simulink model "dynamic_simulation_control"  (R2020b)
settings: Solver=FixedStepAuto  StartTime=time_start  StopTime=time_end  FixedStep=dt  RelTol=1e-3
values from neighbouring files (symbols this model uses):
  B_env = [0;10;0]    [init_dynamic_sim.m]
  dth0 = [0; 0; 0]    [dynamic_simulation.m]    (also in init_dynamic_sim.m = dq0)
  dv = 1e-2    (= 0.01)    [Fs_3DOF.m]    (also in init_dynamic_sim.m)
  Fc = Fs    [Fs_3DOF.m]    (also in init_dynamic_sim.m)
  filt_den = [1/w0^2 2*xi/w0 1]    [init_dynamic_sim.m]
  filt_num = 1    [init_dynamic_sim.m]
  Fs = zeros(3,1)    [DynModel_3DOF.m]    (also in Fs_3DOF.m = [0.97571; 0.65131; 0.25819]; InvDynModel_3DOF.m; init_dynamic_sim.m = [0.97571; 0.65131; 0.25819])
  Fv = zeros(3,3)    [DynModel_3DOF.m]    (also in InvDynModel_3DOF.m; init_dynamic_sim.m = diag([0.5,0.37,0.7]))
  fz0 = 0    [init_dynamic_sim.m]
  K = 0.015    [init_dynamic_sim.m]
  K_env = [0;100;0]    [init_dynamic_sim.m]
  Ki = 0.08    [init_dynamic_sim.m]
  Kj = [1;1;1]*5    [init_dynamic_sim.m]
  Kjd = [1;1;1]*0.1    [init_dynamic_sim.m]
  Kv = [2500;1500;2000]/256    [init_dynamic_sim.m]
  Kvi = [3000;900;1000]/65536    [init_dynamic_sim.m]
  Kx = [20;0;0]    [init_dynamic_sim.m]
  Kxi = [0;0;0]    [init_dynamic_sim.m]
  M_env = [0;1;0]    [init_dynamic_sim.m]
  nu = nu.*eye(3)    [DynModel_3DOF.m]    (also in InvDynModel_3DOF.m; init_dynamic_sim.m = [0.65;0.65;0.65])
  R = [156;100;71]    [init_dynamic_sim.m]
  ry0 = acos(r(1,1))    [init_dynamic_sim.m]
  Tc = [0.0335;0.0335;0.051]    [init_dynamic_sim.m]
  th0 = 0    [DGM_youBot.m]    (also in DGM_youBot_sym.m; dynamic_simulation.m = q_dh - (q0_kuka - q_rob); init_dynamic_sim.m = theta_DH(2:4) - (q0 - KUKA_offset(2:4)))
  thmax = theta_DH - (qmin - KUKA_offset)    [init_dynamic_sim.m]
  thmin = theta_DH - (qmax - KUKA_offset)    [init_dynamic_sim.m]
  x0 = p0(1)    [init_dynamic_sim.m]    (also in jacobian_computation.m = 0.033)
  z0 = 0.3    [dynamic_simulation.m]    (also in init_dynamic_sim.m = p0(3); jacobian_computation.m = 0.147)
undefined symbols (not defined in the file or in its folder): p0
libraries: aerolibutil x1, simulink x1
settings Model: Creator=fortineau_vin  LastModifiedBy=fortineau_vin
settings DataIOCC: ReturnWorkspaceOutputs=off
settings DebuggingCC: ArithmeticOperatorsInVariantConditions=warning
settings SFSimCC: SimUseLocalCustomCode=off  CustomCodeUndefinedFunction=UseInterfaceOnly
settings RTWCC: RTWUseLocalCustomCode=off

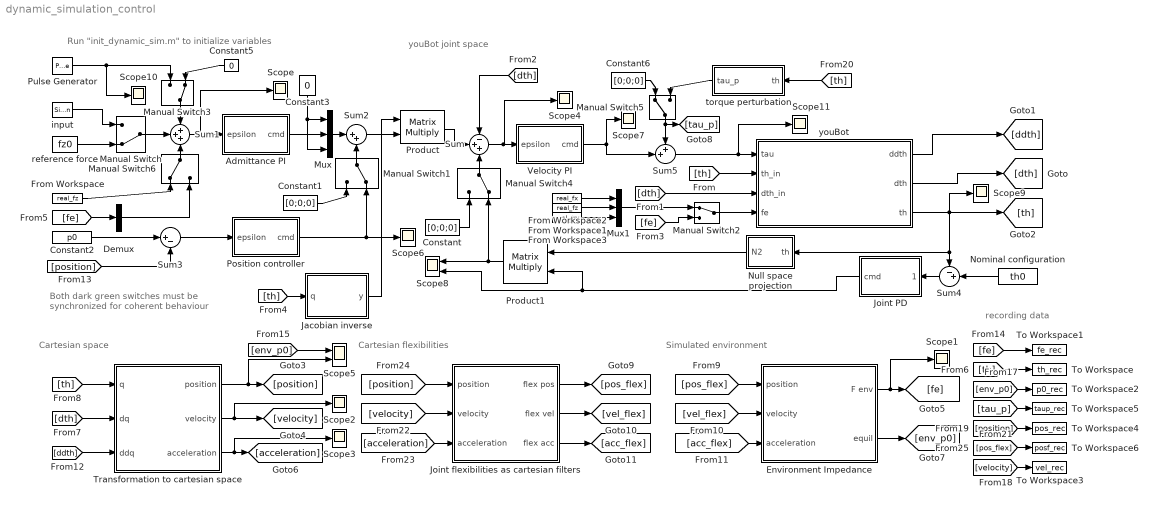
== system dynamic_simulation_control ==
  note: Both dark green switches must
      | be synchronized for coherent behaviour
  note: recording data
  note: Run "init_dynamic_sim.m" to initialize variables
  note: youBot joint space
  note: Simulated environment
  note: Cartesian flexibilities
  note: Cartesian space
  Admittance PI : Subsystem
  Constant : Constant  Value=[0;0;0]
  Constant1 : Constant  Value=[0;0;0]
  Constant2 : Constant  Value=p0
  Constant3 : Constant  Value=0
  Constant5 : Constant  Value=0
  Constant6 : Constant  Value=[0;0;0]
  Demux : Demux  Outputs=3
  "Environment Impedance " : Subsystem
  From Workspace : FromWorkspace  VariableName=real_fz
  From Workspace1 : FromWorkspace  VariableName=real_fz
  From Workspace2 : FromWorkspace  VariableName=real_fx
  From Workspace3 : FromWorkspace  VariableName=real_fry
  Jacobian inverse : MATLAB Function  TreatAsAtomicUnit=on
  Joint PD : Subsystem
  Joint flexibilities as cartesian filters : Subsystem
  Manual Switch{,1,3..4} (4 alike) : ManualSwitch  CurrentSetting=0
  Manual Switch2 : ManualSwitch
  Manual Switch5 : ManualSwitch
  Manual Switch6 : ManualSwitch
  Mux : Mux  Inputs=3
  Mux1 : Mux  Inputs=3
  Nominal configuration : Constant  Value=th0
  Null space projection : Subsystem
  Position controller : Subsystem
  Product : Product  Multiplication=Matrix(*)
  Product1 : Product  Multiplication=Matrix(*)
  Pulse Generator : DiscretePulseGenerator  PulseType=Time based  Amplitude=5  Period=3  PulseWidth=3.3  PhaseDelay=2
  Scope{,1..4,6..7,9..11} (10 alike) : Scope
  Scope5 : Scope  NumInputPorts=2
  Scope8 : Scope  NumInputPorts=2
  Sum : Sum  Inputs=-++
  Sum1 : Sum  Inputs=+++
  Sum2 : Sum  Inputs=|++
  Sum3 : Sum  Inputs=|+-
  Sum4 : Sum  Inputs=-+|
  Sum5 : Sum  Inputs=++|
  To Workspace : ToWorkspace  VariableName=th_rec  SaveFormat=Structure  SampleTime=1e-3
      settings: Save2DSignal=2-D array (concatenate along first dimension)
  To Workspace1 : ToWorkspace  VariableName=fe_rec  SaveFormat=Structure  SampleTime=1e-3
      settings: Save2DSignal=2-D array (concatenate along first dimension)
  To Workspace2 : ToWorkspace  VariableName=p0_rec  SaveFormat=Structure  SampleTime=1e-3
      settings: Save2DSignal=2-D array (concatenate along first dimension)
  To Workspace3 : ToWorkspace  VariableName=vel_rec  SaveFormat=Structure  SampleTime=1e-3
      settings: Save2DSignal=2-D array (concatenate along first dimension)
  To Workspace4 : ToWorkspace  VariableName=pos_rec  SaveFormat=Structure  SampleTime=1e-3
      settings: Save2DSignal=2-D array (concatenate along first dimension)
  To Workspace5 : ToWorkspace  VariableName=taup_rec  SaveFormat=Structure  SampleTime=1e-3
      settings: Save2DSignal=2-D array (concatenate along first dimension)
  To Workspace6 : ToWorkspace  VariableName=posf_rec  SaveFormat=Structure  SampleTime=1e-3
      settings: Save2DSignal=2-D array (concatenate along first dimension)
  Transformation to cartesian space : Subsystem
  Velocity PI : Subsystem
  "input " : SignalGenerator  Amplitude=5  Frequency=0.9  Units=rad/sec
  reference force : Constant  Value=fz0
  torque perturbation : Subsystem
  youBot : Subsystem
  wires:
  Velocity PI/1(cmd) -> Sum5/2, Scope7/1
  Sum/1 -> Scope4/1, Velocity PI/1(epsilon)
  [dth] -> Sum/1
  Product/1 -> Sum/2
  Sum1/1 -> Admittance PI/1(epsilon), Scope/1
  [th] -> Jacobian inverse/1(q)
  [pos_flex] -> "Environment Impedance "/1(position)
  [vel_flex] -> "Environment Impedance "/2(velocity)
  [acc_flex] -> "Environment Impedance "/3(acceleration)
  Position controller/1(cmd) -> Scope6/1, Manual Switch1/2
  Sum3/1 -> Position controller/1(epsilon)
  Constant2/1 -> Sum3/1
  [position] -> Sum3/2
  Admittance PI/1(cmd) -> Mux/2
  Mux/1 -> Sum2/1
  Constant3/1 -> Mux/3, Mux/1
  [th] -> To Workspace/1
  reference force/1 -> Manual Switch/2
  "input "/1 -> Manual Switch/1
  [fe] -> To Workspace1/1
  [th] -> youBot/2(th_in)
  [dth] -> youBot/3(dth_in)
  youBot/1(ddth) -> [ddth]
  youBot/2(dth) -> [dth]
  "Environment Impedance "/2(equil) -> [env_p0]
  Sum4/1 -> Joint PD/1(epsilon)
  Nominal configuration/1 -> Sum4/2
  Product1/1 -> Scope8/1, Manual Switch4/2
  Null space projection/1(N2) -> Product1/1
  youBot/3(th) -> Scope9/1, [th], Null space projection/1(th), Sum4/1
  Joint PD/1(cmd) -> Product1/2, Scope8/2
  Manual Switch4/1 -> Sum/3
  Constant/1 -> Manual Switch4/1
  "Environment Impedance "/1(F env) -> [fe], Scope1/1
  [env_p0] -> To Workspace2/1
  [velocity] -> To Workspace3/1
  [position] -> To Workspace4/1
  Sum2/1 -> Product/2
  Jacobian inverse/1(y) -> Product/1
  Manual Switch1/1 -> Sum2/2
  Constant1/1 -> Manual Switch1/1
  Manual Switch6/1 -> Sum1/3
  Manual Switch/1 -> Sum1/2
  Manual Switch3/1 -> Sum1/1
  Constant5/1 -> Manual Switch3/2
  Pulse Generator/1 -> Scope10/1, Manual Switch3/1
  Sum5/1 -> Scope11/1, youBot/1(tau)
  Manual Switch5/1 -> [tau_p], Sum5/1
  Constant6/1 -> Manual Switch5/1
  torque perturbation/1(tau_p) -> Manual Switch5/2
  [th] -> torque perturbation/1(th)
  [tau_p] -> To Workspace5/1
  [velocity] -> Joint flexibilities as cartesian filters/2(velocity)
  [position] -> Joint flexibilities as cartesian filters/1(position)
  [acceleration] -> Joint flexibilities as cartesian filters/3(acceleration)
  Joint flexibilities as cartesian filters/1(flex pos) -> [pos_flex]
  Joint flexibilities as cartesian filters/2(flex vel) -> [vel_flex]
  Joint flexibilities as cartesian filters/3(flex acc) -> [acc_flex]
  [env_p0] -> Scope5/1
  Transformation to cartesian space/3(acceleration) -> [acceleration], Scope3/1
  Transformation to cartesian space/2(velocity) -> [velocity], Scope2/1
  [th] -> Transformation to cartesian space/1(q)
  [ddth] -> Transformation to cartesian space/3(ddq)
  [dth] -> Transformation to cartesian space/2(dq)
  Transformation to cartesian space/1(position) -> Scope5/2, [position]
  [pos_flex] -> To Workspace6/1
  [fe] -> Demux/1
  From Workspace/1 -> Manual Switch6/1
  Demux/2 -> Manual Switch6/2
  Mux1/1 -> Manual Switch2/1
  From Workspace1/1 -> Mux1/2
  [fe] -> Manual Switch2/2
  From Workspace2/1 -> Mux1/1
  From Workspace3/1 -> Mux1/3
  Manual Switch2/1 -> youBot/4(fe)

== system dynamic_simulation_control/Admittance PI ==
  epsilon : Inport
  Gain : Gain  Gain=K
  Gain1 : Gain  Gain=Ki
  Integrator2 : Integrator
  Sum : Sum  Inputs=|++
  cmd : Outport  VectorParamsAs1DForOutWhenUnconnected=off
  wires:
  Integrator2/1 -> Sum/2
  Gain/1 -> Sum/1
  Gain1/1 -> Integrator2/1
  epsilon/1 -> Gain/1, Gain1/1
  Sum/1 -> cmd/1

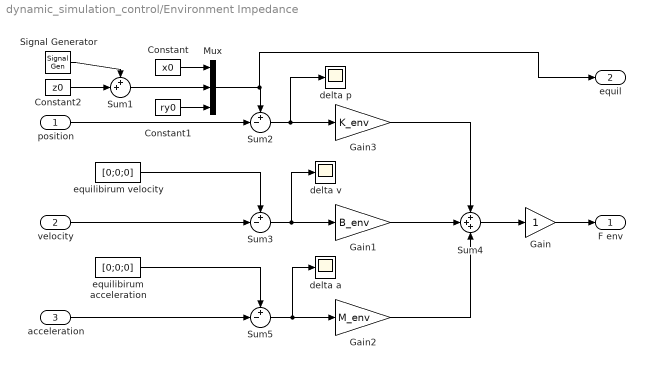
== system dynamic_simulation_control/Environment Impedance  ==
  position : Inport
  velocity : Inport  Port=2
  acceleration : Inport  Port=3
  Constant : Constant  Value=x0
  Constant1 : Constant  Value=ry0
  Constant2 : Constant  Value=z0
  Gain : Gain
  Gain1 : Gain  Gain=B_env
  Gain2 : Gain  Gain=M_env
  Gain3 : Gain  Gain=K_env
  Mux : Mux  Inputs=3
  Signal Generator : SignalGenerator  Amplitude=0.03  Frequency=0.9
  Sum1 : Sum  Inputs=++|
  Sum2 : Sum  Inputs=+-|
  Sum3 : Sum  Inputs=+-|
  Sum4 : Sum  Inputs=+++
  Sum5 : Sum  Inputs=+-|
  delta a : Scope
  delta p : Scope
  delta v : Scope
  equilibirum acceleration : Constant  Value=[0;0;0]
  equilibirum velocity : Constant  Value=[0;0;0]
  F env : Outport  VectorParamsAs1DForOutWhenUnconnected=off
  equil : Outport  Port=2  VectorParamsAs1DForOutWhenUnconnected=off
  wires:
  Gain3/1 -> Sum4/1
  velocity/1 -> Sum3/2
  position/1 -> Sum2/2
  Gain2/1 -> Sum4/3
  equilibirum velocity/1 -> Sum3/1
  Sum3/1 -> delta v/1, Gain1/1
  Sum4/1 -> Gain/1
  acceleration/1 -> Sum5/2
  Sum5/1 -> delta a/1, Gain2/1
  Gain1/1 -> Sum4/2
  equilibirum acceleration/1 -> Sum5/1
  Sum2/1 -> delta p/1, Gain3/1
  Constant/1 -> Mux/1
  Constant1/1 -> Mux/3
  Mux/1 -> equil/1, Sum2/1
  Sum1/1 -> Mux/2
  Constant2/1 -> Sum1/2
  Signal Generator/1 -> Sum1/1
  Gain/1 -> F env/1

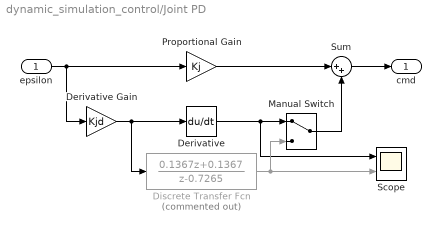
== system dynamic_simulation_control/Joint PD ==
  epsilon : Inport
  " Derivative Gain" : Gain  Gain=Kjd
  Derivative : Derivative
  Discrete Transfer Fcn : DiscreteTransferFcn  Commented=on  Numerator=[0.1367 0.1367]  Denominator=[1 -0.7265]
  Manual Switch : ManualSwitch
  Proportional Gain : Gain  Gain=Kj
  Scope : Scope  NumInputPorts=2
  Sum : Sum  Inputs=|++
  cmd : Outport  VectorParamsAs1DForOutWhenUnconnected=off
  wires:
  Sum/1 -> cmd/1
  epsilon/1 -> " Derivative Gain"/1, Proportional Gain/1
  " Derivative Gain"/1 -> Derivative/1, Discrete Transfer Fcn/1
  Proportional Gain/1 -> Sum/1
  Derivative/1 -> Scope/1, Manual Switch/1
  Manual Switch/1 -> Sum/2
  Discrete Transfer Fcn/1 -> Scope/2, Manual Switch/2

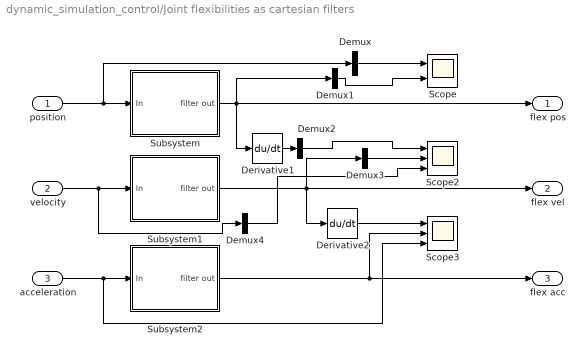
== system dynamic_simulation_control/Joint flexibilities as cartesian filters ==
  position : Inport
  velocity : Inport  Port=2
  acceleration : Inport  Port=3
  Demux{,1..4} (5 alike) : Demux  Outputs=3
  Derivative1 : Derivative
  Derivative2 : Derivative
  Scope : Scope  NumInputPorts=2
  Scope2 : Scope  NumInputPorts=3
  Scope3 : Scope  NumInputPorts=3
  Subsystem : Subsystem
  Subsystem1 : Subsystem
  Subsystem2 : Subsystem
  flex pos : Outport  VectorParamsAs1DForOutWhenUnconnected=off
  flex vel : Outport  Port=2  VectorParamsAs1DForOutWhenUnconnected=off
  flex acc : Outport  Port=3  VectorParamsAs1DForOutWhenUnconnected=off
  wires:
  Subsystem/1(filter out) -> Demux1/1, Derivative1/1, flex pos/1
  position/1 -> Demux/1, Subsystem/1(In)
  velocity/1 -> Demux4/1, Subsystem1/1(In)
  Subsystem1/1(filter out) -> Demux3/1, flex vel/1, Derivative2/1
  acceleration/1 -> Scope3/3, Subsystem2/1(In)
  Subsystem2/1(filter out) -> Scope3/2, flex acc/1
  Derivative2/1 -> Scope3/1
  Demux/2 -> Scope/1
  Demux1/2 -> Scope/2
  Derivative1/1 -> Demux2/1
  Demux2/2 -> Scope2/1
  Demux3/2 -> Scope2/2
  Demux4/2 -> Scope2/3

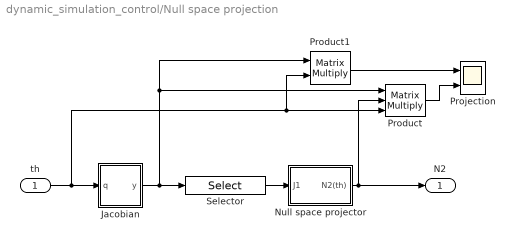
== system dynamic_simulation_control/Null space projection ==
  th : Inport
  Jacobian : MATLAB Function  TreatAsAtomicUnit=on
  Null space projector : Subsystem
  Product : Product  Inputs=3  Multiplication=Matrix(*)
  Product1 : Product  Multiplication=Matrix(*)
  Projection : Scope  NumInputPorts=2
  Selector : Selector  NumberOfDimensions=2  InputPortWidth=3  IndexOptions=Index vector (dialog),Index vector (dialog)  Indices=2,[1 2 3]  OutputSizes=1,1
  N2 : Outport  VectorParamsAs1DForOutWhenUnconnected=off
  wires:
  Null space projector/1(N2(th)) -> N2/1, Product/2
  Jacobian/1(y) -> Product1/1, Product/1, Selector/1
  Selector/1 -> Null space projector/1(J1)
  th/1 -> Product1/2, Product/3, Jacobian/1(q)
  Product/1 -> Projection/2
  Product1/1 -> Projection/1

== system dynamic_simulation_control/Position controller ==
  epsilon : Inport
  Gain : Gain  Gain=Kx
  Gain1 : Gain  Gain=Kxi
  Integrator2 : Integrator
  Sum : Sum  Inputs=|++
  cmd : Outport  VectorParamsAs1DForOutWhenUnconnected=off
  wires:
  Sum/1 -> cmd/1
  epsilon/1 -> Gain1/1, Gain/1
  Gain1/1 -> Integrator2/1
  Gain/1 -> Sum/1
  Integrator2/1 -> Sum/2

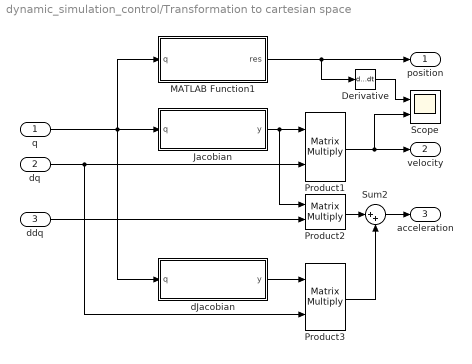
== system dynamic_simulation_control/Transformation to cartesian space ==
  q : Inport
  dq : Inport  Port=2
  ddq : Inport  Port=3
  Derivative : Derivative
  Jacobian : MATLAB Function  TreatAsAtomicUnit=on
  MATLAB Function1 : MATLAB Function  TreatAsAtomicUnit=on
  Product1 : Product  Multiplication=Matrix(*)
  Product2 : Product  Multiplication=Matrix(*)
  Product3 : Product  Multiplication=Matrix(*)
  Scope : Scope  NumInputPorts=2
  Sum2 : Sum  Inputs=|++
  dJacobian : MATLAB Function  TreatAsAtomicUnit=on
  position : Outport  VectorParamsAs1DForOutWhenUnconnected=off
  velocity : Outport  Port=2  VectorParamsAs1DForOutWhenUnconnected=off
  acceleration : Outport  Port=3  VectorParamsAs1DForOutWhenUnconnected=off
  wires:
  MATLAB Function1/1(res) -> Derivative/1, position/1
  q/1 -> dJacobian/1(q), MATLAB Function1/1(q), Jacobian/1(q)
  Product1/1 -> Scope/2, velocity/1
  Product2/1 -> Sum2/1
  Sum2/1 -> acceleration/1
  Product3/1 -> Sum2/2
  dq/1 -> Product3/2, Product1/2
  Jacobian/1(y) -> Product2/1, Product1/1
  ddq/1 -> Product2/2
  dJacobian/1(y) -> Product3/1
  Derivative/1 -> Scope/1

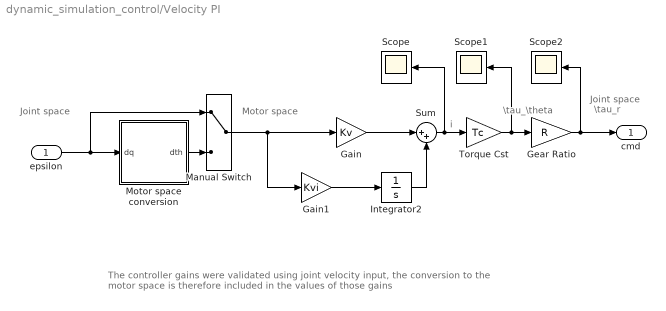
== system dynamic_simulation_control/Velocity PI ==
  note: The controller gains were validated using joint velocity input, the conversion to
      | the motor space is therefore included in the values of those gains
  note: \tau_\theta
  note: i
  note: Motor space
  note: Joint space
  note: \tau_r
  note: Joint space
  epsilon : Inport
  Gain : Gain  Gain=Kv
  Gain1 : Gain  Gain=Kvi
  Gear Ratio : Gain  Gain=R
  Integrator2 : Integrator
  Manual Switch : ManualSwitch
  Motor space conversion : Subsystem
  Scope : Scope
  Scope1 : Scope
  Scope2 : Scope
  Sum : Sum  Inputs=|++
  Torque Cst : Gain  Gain=Tc
  cmd : Outport  VectorParamsAs1DForOutWhenUnconnected=off
  wires:
  Gain1/1 -> Integrator2/1
  Gain/1 -> Sum/1
  Integrator2/1 -> Sum/2
  Gear Ratio/1 -> Scope2/1, cmd/1
  Sum/1 -> Scope/1, Torque Cst/1
  Torque Cst/1 -> Scope1/1, Gear Ratio/1
  epsilon/1 -> Manual Switch/1, Motor space conversion/1(dq)
  Motor space conversion/1(dth) -> Manual Switch/2
  Manual Switch/1 -> Gain1/1, Gain/1

== system dynamic_simulation_control/torque perturbation ==
  note: joint space
  note: force perturbation on z axis
  th : Inport
  Constant : Constant  Value=0
  MATLAB Function2 : MATLAB Function  TreatAsAtomicUnit=on
  Mux : Mux  Inputs=3
  Product : Product  Multiplication=Matrix(*)
  Pulse Generator1 : DiscretePulseGenerator  PulseType=Time based  Amplitude=10  Period=3  PhaseDelay=2
  tau_p : Outport  VectorParamsAs1DForOutWhenUnconnected=off
  wires:
  Pulse Generator1/1 -> Mux/2
  Constant/1 -> Mux/1, Mux/3
  th/1 -> MATLAB Function2/1(q)
  MATLAB Function2/1(y) -> Product/1
  Mux/1 -> Product/2
  Product/1 -> tau_p/1

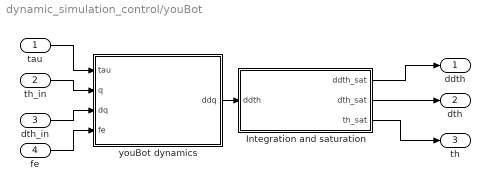
== system dynamic_simulation_control/youBot ==
  tau : Inport
  th_in : Inport  Port=2
  dth_in : Inport  Port=3
  fe : Inport  Port=4
  Integration and saturation : Subsystem
  youBot dynamics : Subsystem
  ddth : Outport  VectorParamsAs1DForOutWhenUnconnected=off
  dth : Outport  Port=2  VectorParamsAs1DForOutWhenUnconnected=off
  th : Outport  Port=3  VectorParamsAs1DForOutWhenUnconnected=off
  wires:
  tau/1 -> youBot dynamics/1(tau)
  youBot dynamics/1(ddq) -> Integration and saturation/1(ddth)
  dth_in/1 -> youBot dynamics/3("dq ")
  th_in/1 -> youBot dynamics/2("q ")
  fe/1 -> youBot dynamics/4(fe)
  Integration and saturation/3(th_sat) -> th/1
  Integration and saturation/1(ddth_sat) -> ddth/1
  Integration and saturation/2(dth_sat) -> dth/1

== system dynamic_simulation_control/Joint flexibilities as cartesian filters/Subsystem ==
  In : Inport
  Demux : Demux  Outputs=3
  Mux : Mux  Inputs=3
  Transfer Fcn : TransferFcn  Numerator=filt_num  Denominator=filt_den
  Transfer Fcn1 : TransferFcn  Numerator=filt_num  Denominator=filt_den
  Transfer Fcn2 : TransferFcn  Numerator=filt_num  Denominator=filt_den
  filter out : Outport  VectorParamsAs1DForOutWhenUnconnected=off
  wires:
  Demux/2 -> Transfer Fcn/1
  In/1 -> Demux/1
  Demux/3 -> Transfer Fcn1/1
  Demux/1 -> Transfer Fcn2/1
  Transfer Fcn2/1 -> Mux/1
  Transfer Fcn/1 -> Mux/2
  Transfer Fcn1/1 -> Mux/3
  Mux/1 -> filter out/1

== system dynamic_simulation_control/Joint flexibilities as cartesian filters/Subsystem1 ==
  In : Inport
  Demux : Demux  Outputs=3
  Mux : Mux  Inputs=3
  Transfer Fcn : TransferFcn  Numerator=filt_num  Denominator=filt_den
  Transfer Fcn1 : TransferFcn  Numerator=filt_num  Denominator=filt_den
  Transfer Fcn2 : TransferFcn  Numerator=filt_num  Denominator=filt_den
  filter out : Outport  VectorParamsAs1DForOutWhenUnconnected=off
  wires:
  Demux/2 -> Transfer Fcn/1
  In/1 -> Demux/1
  Demux/3 -> Transfer Fcn1/1
  Demux/1 -> Transfer Fcn2/1
  Transfer Fcn2/1 -> Mux/1
  Transfer Fcn/1 -> Mux/2
  Transfer Fcn1/1 -> Mux/3
  Mux/1 -> filter out/1

== system dynamic_simulation_control/Joint flexibilities as cartesian filters/Subsystem2 ==
  In : Inport
  Demux : Demux  Outputs=3
  Mux : Mux  Inputs=3
  Transfer Fcn : TransferFcn  Numerator=filt_num  Denominator=filt_den
  Transfer Fcn1 : TransferFcn  Numerator=filt_num  Denominator=filt_den
  Transfer Fcn2 : TransferFcn  Numerator=filt_num  Denominator=filt_den
  filter out : Outport  VectorParamsAs1DForOutWhenUnconnected=off
  wires:
  Demux/2 -> Transfer Fcn/1
  In/1 -> Demux/1
  Demux/3 -> Transfer Fcn1/1
  Demux/1 -> Transfer Fcn2/1
  Transfer Fcn2/1 -> Mux/1
  Transfer Fcn/1 -> Mux/2
  Transfer Fcn1/1 -> Mux/3
  Mux/1 -> filter out/1

== system dynamic_simulation_control/Null space projection/Null space projector ==
  J1 : Inport
  Constant : Constant  Value=eye(3)  VectorParams1D=off
  Constant1 : Constant  Value=eye(3)  VectorParams1D=off
  Product : Product  Multiplication=Matrix(*)
  Pseudo inverse : Subsystem
  Sum : Sum  Inputs=|+-
  N2(th) : Outport  VectorParamsAs1DForOutWhenUnconnected=off
  wires:
  Constant/1 -> Sum/1
  Constant1/1 -> Pseudo inverse/2(W)
  J1/1 -> Pseudo inverse/1(A), Product/2
  Pseudo inverse/1(A^W+) -> Product/1
  Product/1 -> Sum/2
  Sum/1 -> N2(th)/1

== system dynamic_simulation_control/Velocity PI/Motor space conversion ==
  note: motor space
  note: turn per minute
  dq : Inport
  Gain1 : Gain  Gain=60/(2*pi)
  Gear ratio : Gain  Gain=R
  dth : Outport  VectorParamsAs1DForOutWhenUnconnected=off
  wires:
  dq/1 -> Gear ratio/1
  Gear ratio/1 -> Gain1/1
  Gain1/1 -> dth/1

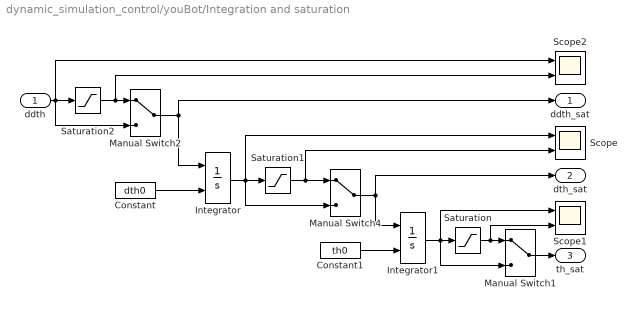
== system dynamic_simulation_control/youBot/Integration and saturation ==
  ddth : Inport
  Constant : Constant  Value=dth0
  Constant1 : Constant  Value=th0
  Integrator : Integrator  InitialConditionSource=external
  Integrator1 : Integrator  InitialConditionSource=external
  Manual Switch1 : ManualSwitch
  Manual Switch2 : ManualSwitch
  Manual Switch4 : ManualSwitch
  Saturation : Saturate  UpperLimit=thmax(2:4)'  LowerLimit=thmin(2:4)'
  Saturation1 : Saturate  UpperLimit=[2.685122; 4.188790; 5.899705]  LowerLimit=[-2.685122; -4.188790; -5.899705]
  Saturation2 : Saturate  UpperLimit=[10;10;10]  LowerLimit=[-10;-10;-10]
  Scope : Scope  NumInputPorts=2
  Scope1 : Scope  NumInputPorts=2
  Scope2 : Scope  NumInputPorts=2
  ddth_sat : Outport  VectorParamsAs1DForOutWhenUnconnected=off
  dth_sat : Outport  Port=2  VectorParamsAs1DForOutWhenUnconnected=off
  th_sat : Outport  Port=3  VectorParamsAs1DForOutWhenUnconnected=off
  wires:
  Manual Switch2/1 -> ddth_sat/1, Integrator/1
  Manual Switch1/1 -> th_sat/1
  Manual Switch4/1 -> Integrator1/1, dth_sat/1
  ddth/1 -> Scope2/1, Manual Switch2/2, Saturation2/1
  Saturation2/1 -> Scope2/2, Manual Switch2/1
  Saturation1/1 -> Scope/2, Manual Switch4/1
  Saturation/1 -> Scope1/2, Manual Switch1/1
  Constant/1 -> Integrator/2
  Integrator/1 -> Scope/1, Manual Switch4/2, Saturation1/1
  Integrator1/1 -> Scope1/1, Manual Switch1/2, Saturation/1
  Constant1/1 -> Integrator1/2

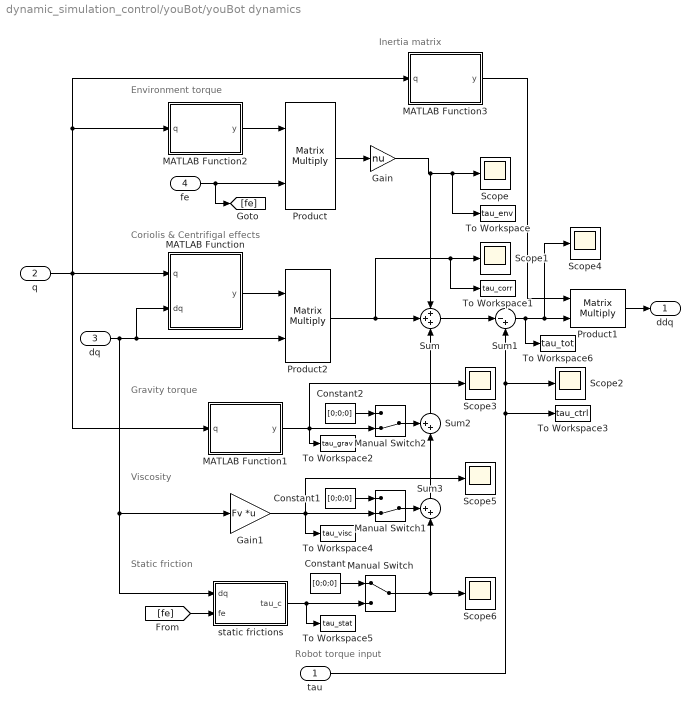
== system dynamic_simulation_control/youBot/youBot dynamics ==
  note: Coriolis & Centrifigal effects
  note: Gravity torque
  note: Environment torque
  note: Robot torque input
  note: Inertia matrix
  note: Viscosity
  note: Static friction
  tau : Inport
  "q " : Inport  Port=2
  "dq " : Inport  Port=3
  fe : Inport  Port=4
  Constant : Constant  Value=[0;0;0]
  Constant1 : Constant  Value=[0;0;0]
  Constant2 : Constant  Value=[0;0;0]
  Gain : Gain  Gain=nu
  Gain1 : Gain  Gain=Fv  Multiplication=Matrix(K*u)
  MATLAB Function : MATLAB Function  TreatAsAtomicUnit=on
  MATLAB Function1 : MATLAB Function  TreatAsAtomicUnit=on
  MATLAB Function2 : MATLAB Function  TreatAsAtomicUnit=on
  MATLAB Function3 : MATLAB Function  TreatAsAtomicUnit=on
  Manual Switch : ManualSwitch
  Manual Switch1 : ManualSwitch  CurrentSetting=0
  Manual Switch2 : ManualSwitch  CurrentSetting=0
  Product : Product  Multiplication=Matrix(*)
  Product1 : Product  Multiplication=Matrix(*)
  Product2 : Product  Multiplication=Matrix(*)
  Scope{,1..6} (7 alike) : Scope
  Sum : Sum  Inputs=+++
  Sum1 : Sum  Inputs=|-+
  Sum2 : Sum  Inputs=++|
  Sum3 : Sum  Inputs=++|
  To Workspace : ToWorkspace  VariableName=tau_env  SaveFormat=Timeseries  SampleTime=-1
  To Workspace1 : ToWorkspace  VariableName=tau_corr  SaveFormat=Timeseries  SampleTime=-1
  To Workspace2 : ToWorkspace  VariableName=tau_grav  SaveFormat=Timeseries  SampleTime=-1
  To Workspace3 : ToWorkspace  VariableName=tau_ctrl  SaveFormat=Timeseries  SampleTime=-1
  To Workspace4 : ToWorkspace  VariableName=tau_visc  SaveFormat=Timeseries  SampleTime=-1
  To Workspace5 : ToWorkspace  VariableName=tau_stat  SaveFormat=Timeseries  SampleTime=-1
  To Workspace6 : ToWorkspace  VariableName=tau_tot  SaveFormat=Timeseries  SampleTime=-1
  static frictions : Subsystem
  ddq : Outport  VectorParamsAs1DForOutWhenUnconnected=off
  wires:
  "dq "/1 -> Product2/2, MATLAB Function/2(dq), static frictions/1(dq), Gain1/1
  "q "/1 -> MATLAB Function/1(q), MATLAB Function2/1(q), MATLAB Function3/1(q), MATLAB Function1/1(q)
  Product/1 -> Gain/1
  Product1/1 -> ddq/1
  MATLAB Function1/1(y) -> Scope3/1, Manual Switch2/2, To Workspace2/1
  Sum/1 -> Sum1/1
  Product2/1 -> Scope1/1, To Workspace1/1, Sum/2
  MATLAB Function/1(y) -> Product2/1
  MATLAB Function2/1(y) -> Product/1
  fe/1 -> Product/2, [fe]
  MATLAB Function3/1(y) -> Product1/1
  Sum1/1 -> To Workspace6/1, Scope4/1, Product1/2
  tau/1 -> To Workspace3/1, Scope2/1, Sum1/2
  Gain/1 -> Scope/1, To Workspace/1, Sum/1
  Sum2/1 -> Sum/3
  Gain1/1 -> Manual Switch1/2, Scope5/1, To Workspace4/1
  [fe] -> static frictions/2(fe)
  Sum3/1 -> Sum2/2
  static frictions/1(tau_c) -> To Workspace5/1, Manual Switch/2
  Manual Switch/1 -> Sum3/2, Scope6/1
  Constant/1 -> Manual Switch/1
  Constant1/1 -> Manual Switch1/1
  Manual Switch1/1 -> Sum3/1
  Manual Switch2/1 -> Sum2/1
  Constant2/1 -> Manual Switch2/1

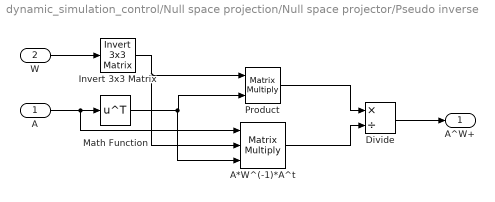
== system dynamic_simulation_control/Null space projection/Null space projector/Pseudo inverse ==
  A : Inport
  W : Inport  Port=2
  A*W^(-1)*A^t : Product  Inputs=3  Multiplication=Matrix(*)
  Divide : Product  Inputs=*/
  Invert 3x3 Matrix : aerolibutil/Invert  3x3 Matrix
  Math Function : Math  Operator=transpose  SignedPower=on  SaturateOnIntegerOverflow=on
  Product : Product  Multiplication=Matrix(*)
  A^W+ : Outport  VectorParamsAs1DForOutWhenUnconnected=off
  wires:
  W/1 -> Invert 3x3 Matrix/1
  A/1 -> A*W^(-1)*A^t/1, Math Function/1
  Math Function/1 -> A*W^(-1)*A^t/3, Product/2
  Invert 3x3 Matrix/1 -> A*W^(-1)*A^t/2, Product/1
  Product/1 -> Divide/1
  A*W^(-1)*A^t/1 -> Divide/2
  Divide/1 -> A^W+/1

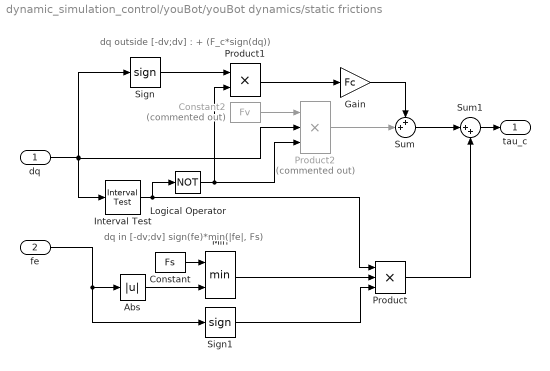
== system dynamic_simulation_control/youBot/youBot dynamics/static frictions ==
  note: dq in [-dv;dv]
      |
      | sign(fe)*min(|fe|, Fs)
  note: dq outside [-dv;dv] : + (F_c*sign(dq))
  dq : Inport
  fe : Inport  Port=2
  Abs : Abs
  Constant : Constant  Value=Fs
  Constant2 : Constant  Commented=on  Value=Fv
  Gain : Gain  Gain=Fc
  Interval Test : simulink/Logic and Bit Operations/Interval Test  IntervalClosedRight=on  uplimit=dv  IntervalClosedLeft=on  lowlimit=-dv  OutDataTypeStr=boolean
  Logical Operator : Logic  Operator=NOT  AllPortsSameDT=off  OutDataTypeStr=boolean
  Min : MinMax  Inputs=2
  Product : Product  Inputs=3
  Product1 : Product
  Product2 : Product  Commented=on  Inputs=3
  Sign : Signum
  Sign1 : Signum
  Sum : Sum  Inputs=++|
  Sum1 : Sum  Inputs=|++
  tau_c : Outport  VectorParamsAs1DForOutWhenUnconnected=off
  wires:
  Sum1/1 -> tau_c/1
  Interval Test/1 -> Logical Operator/1, Product/1
  fe/1 -> Sign1/1, Abs/1
  Abs/1 -> Min/2
  Constant/1 -> Min/1
  Min/1 -> Product/2
  Sign1/1 -> Product/3
  Logical Operator/1 -> Product1/2, Product2/3
  dq/1 -> Sign/1, Product2/2, Interval Test/1
  Constant2/1 -> Product2/1
  Product2/1 -> Sum/2
  Product1/1 -> Gain/1
  Sum/1 -> Sum1/1
  Product/1 -> Sum1/2
  Sign/1 -> Product1/1
  Gain/1 -> Sum/1

== matlab function dynamic_simulation_control/youBot/youBot dynamics/MATLAB Function ==
  data: q input; y output; dq input
function y = C_sim(q,dq)
q2 = q(2);
q3 = q(3);
dq1 = dq(1);
dq2 = dq(2);
dq3 = dq(3);
y = C_3DOF(dq1,dq2,dq3,q2,q3);

== matlab function dynamic_simulation_control/youBot/youBot dynamics/MATLAB Function2 ==
  data: q input; y output
function y = tJ_sim(q)
q1 = q(1);
q2 = q(2);
q3 = q(3);
y = J0E_3DOF(q1,q2,q3)';

== matlab function dynamic_simulation_control/youBot/youBot dynamics/MATLAB Function3 ==
  data: q input; y output
function y = iM_sim(q)
q2 = q(2);
q3 = q(3);
y = iM_3DOF(q2,q3);

== matlab function dynamic_simulation_control/Jacobian inverse ==
  data: q input; y output
function y = iJ(q)
q1 = q(1);
q2 = q(2);
q3 = q(3);
y = iJ0E_3DOF(q1,q2,q3);

== matlab function dynamic_simulation_control/Transformation to cartesian space/dJacobian ==
  data: q input; y output
function y = dJ(q)
q1 = q(1);
q2 = q(2);
q3 = q(3);
y = dJ0E_3DOF(q1,q2,q3);

== matlab function dynamic_simulation_control/Transformation to cartesian space/Jacobian ==
  data: q input; y output
function y = J(q)
q1 = q(1);
q2 = q(2);
q3 = q(3);
y = J0E_3DOF(q1,q2,q3);

== matlab function dynamic_simulation_control/Transformation to cartesian space/MATLAB Function1 ==
  data: q input; res output
function res = forwardKinematics(q)

x0 = 0;
le = 0.1;

[p,r,~] = DGM_youBot(q, x0, le);

x  = p(1);
z  = p(3);
ry = acos(r(1,1));

res = [x,z,ry]';

== matlab function dynamic_simulation_control/Null space projection/Jacobian ==
  data: q input; y output
function y = J(q)
q1 = q(1);
q2 = q(2);
q3 = q(3);
y = J0E_3DOF(q1,q2,q3);

== matlab function dynamic_simulation_control/torque perturbation/MATLAB Function2 ==
  data: q input; y output
function y = tJ_sim(q)
q1 = q(1);
q2 = q(2);
q3 = q(3);
y = J0E_3DOF(q1,q2,q3)';

== matlab function dynamic_simulation_control/youBot/youBot dynamics/MATLAB Function1 ==
  data: q input; y output
function y = G_sim(q)
q1 = q(1);
q2 = q(2);
q3 = q(3);
y = G_3DOF(q1,q2,q3);
